simulink model "boost9_non_ideal"  (R2020a)
settings: Solver=VariableStepAuto  StartTime=0.0  StopTime=0.3  RelTol=1e-3
libraries: powerlib x16, powerlib_meascontrol x4
settings Model: Creator=Admin  LastModifiedBy=Admin

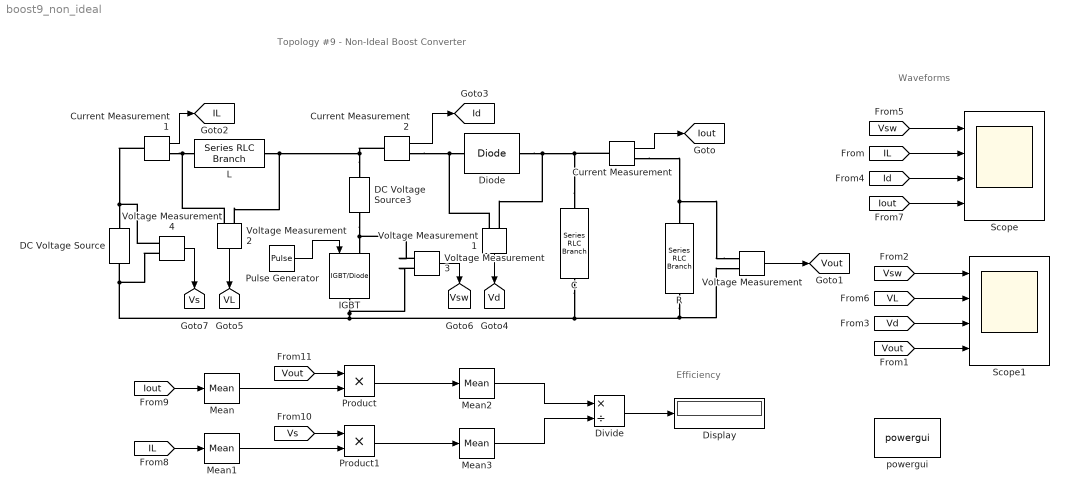
== system boost9_non_ideal ==
  note: Waveforms
  note: Topology #9 - Non-Ideal Boost Converter
  note: Efficiency
  C : powerlib/Elements/Series RLC Branch  LConnTagsString=__new0  RConnTagsString=__new0  BranchType=C  Resistance=1  Inductance=1e-3  SetiL0=off  InitialCurrent=0  Capacitance=0.0000074  Setx0=off  InitialVoltage=0  Measurements=None
  Current Measurement : powerlib/Measurements/Current Measurement  PhasorSimulation=off  OutputType=Complex  PSBequivalent=0
  Current Measurement1 : powerlib/Measurements/Current Measurement  PhasorSimulation=off  OutputType=Complex  PSBequivalent=0
  Current Measurement2 : powerlib/Measurements/Current Measurement  PhasorSimulation=off  OutputType=Complex  PSBequivalent=0
  DC Voltage Source : powerlib/Electrical Sources/DC Voltage Source  Amplitude=36  Measurements=Voltage
      settings: AttributesFormatString=%<Amplitude>
  DC Voltage Source3 : powerlib/Electrical Sources/DC Voltage Source  Amplitude=0.9  Measurements=Voltage
      settings: AttributesFormatString=%<Amplitude>
  Diode : powerlib/Power Electronics/Diode  Ron=0  Lon=0  Vf=0.5  IC=0  UseSnubber=off  Rs=inf  Cs=0  Measurements=off
  Display : Display
  Divide : Product  Inputs=*/
  IGBT : powerlib/Power Electronics/IGBT//Diode  Ron=1e-3  Rs=1e5  Cs=inf  Measurements=off
  L : powerlib/Elements/Series RLC Branch  LConnTagsString=__new0  RConnTagsString=__new0  BranchType=L  Resistance=1  Inductance=0.00653  SetiL0=on  InitialCurrent=0  Capacitance=1e-6  Setx0=off  InitialVoltage=0  Measurements=Branch current
  Mean : powerlib_meascontrol/Measurements/Mean  Freq=20000  Vinit=0  Ts=0
  Mean1 : powerlib_meascontrol/Measurements/Mean  Freq=20000  Vinit=0  Ts=0
  Mean2 : powerlib_meascontrol/Measurements/Mean  Freq=60  Vinit=0  Ts=0
  Mean3 : powerlib_meascontrol/Measurements/Mean  Freq=60  Vinit=0  Ts=0
  Product : Product
  Product1 : Product
  Pulse Generator : DiscretePulseGenerator  PulseType=Time based  Period=1/20000  PulseWidth=60
  R : powerlib/Elements/Series RLC Branch  LConnTagsString=__new0  RConnTagsString=__new0  BranchType=R  Resistance=140  Inductance=1e-3  SetiL0=off  InitialCurrent=0  Capacitance=1e-6  Setx0=off  InitialVoltage=0  Measurements=None
  Scope : Scope  NumInputPorts=4
  Scope1 : Scope  NumInputPorts=4
  Voltage Measurement{,1..4} (5 alike) : powerlib/Measurements/Voltage Measurement  PhasorSimulation=off  OutputType=Complex  PSBequivalent=0
  powergui : powerlib/powergui  Priority=1  SimulationMode=Continuous  SampleTime=50e-6  frequency=60  Iterations=50  frequencyindice=0  Pbase=100e6  ErrMax=1e-4  UnitsV=kV  UnitsW=MW  buscounter=0  FunctionMessages=off  echomessages=off  EnableUseOfTLC=off  CurrentSourceSwitches=off  DisableSnubberDevices=off  DisableRonSwitches=off  DisableVfSwitches=off  DisplayEquations=off  AutomaticDiscreteSolvers=off  SolverType=Tustin/Backward Euler (TBE)  Interpol=off  ExternalGateDelay=off  methode=off  Ts=100  x0status=blocks  SPID=off  SwTol=0  HookPort=off  NonlinearTolerance=1e-4  nMaxIteration=100  ContinueOnMaxIteration=off  RestoreLinks=warning  ResistiveCurrentMeasurement=off  Frange=[0:2:500]  Ylog=off  Xlog=on  ShowGrid=off  save=off  variable=ZData  structure=0  ZoomFFT=off  StartTime=0.0  cycles=1  DisplayStyle=1  fundamental=60  FreqAxis=off  MaxFrequency=1000  frequencyindicesteady=1  RmsSteady=1  display=off
  tag scope: IL=global, Id=global, Iout=global, VL=global, Vd=global, Vout=global, Vs=global, Vsw=global
  wires:
  [Vsw] -> Scope/1
  [Vout] -> Scope1/4
  [Id] -> Scope/3
  Current Measurement/1 -> [Iout]
  Current Measurement1/1 -> [IL]
  Voltage Measurement1/1 -> [Vd]
  Voltage Measurement3/1 -> [Vsw]
  Voltage Measurement2/1 -> [VL]
  Voltage Measurement/1 -> [Vout]
  [Vd] -> Scope1/3
  Current Measurement2/1 -> [Id]
  Pulse Generator/1 -> IGBT/1
  [Iout] -> Scope/4
  [Vsw] -> Scope1/1
  [IL] -> Scope/2
  [VL] -> Scope1/2
  Mean2/1 -> Divide/1
  Divide/1 -> Display/1
  Mean3/1 -> Divide/2
  Mean1/1 -> Product1/2
  [Iout] -> Mean/1
  Product/1 -> Mean2/1
  [Vout] -> Product/1
  [Vs] -> Product1/1
  Product1/1 -> Mean3/1
  [IL] -> Mean1/1
  Mean/1 -> Product/2
  Voltage Measurement4/1 -> [Vs]
  connections:
  L/LConn1 -- Current Measurement1/RConn1 -- Voltage Measurement2/LConn1
  Diode/LConn1 -- Current Measurement2/RConn1 -- Voltage Measurement1/LConn1
  C/LConn1 -- Current Measurement/LConn1 -- Diode/RConn1 -- Voltage Measurement1/LConn2
  IGBT/RConn1 -- Voltage Measurement3/LConn2 -- R/RConn1 -- Voltage Measurement/LConn2 -- C/RConn1 -- Voltage Measurement4/LConn2 -- DC Voltage Source/LConn1
  Voltage Measurement/LConn1 -- Current Measurement/RConn1 -- R/LConn1
  DC Voltage Source3/RConn1 -- L/RConn1 -- Voltage Measurement2/LConn2 -- Current Measurement2/LConn1
  Current Measurement1/LConn1 -- DC Voltage Source/RConn1 -- Voltage Measurement4/LConn1
  DC Voltage Source3/LConn1 -- Voltage Measurement3/LConn1 -- IGBT/LConn1
